simulink model "sampleModel1582_2"  (R2023a)
settings: Solver=VariableStepAuto  StartTime=0.0  StopTime=10.0  RelTol=1e-3
libraries: simulink x4, hdlsllib x1
settings Model: Creator=user1  LastModifiedBy=user1

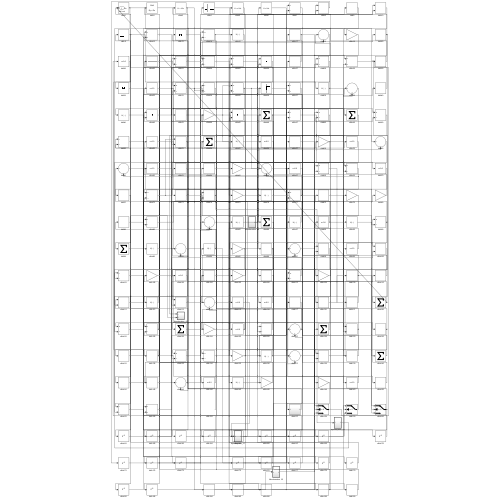
[thumbnail: Simulink's stored preview of the top-level diagram]
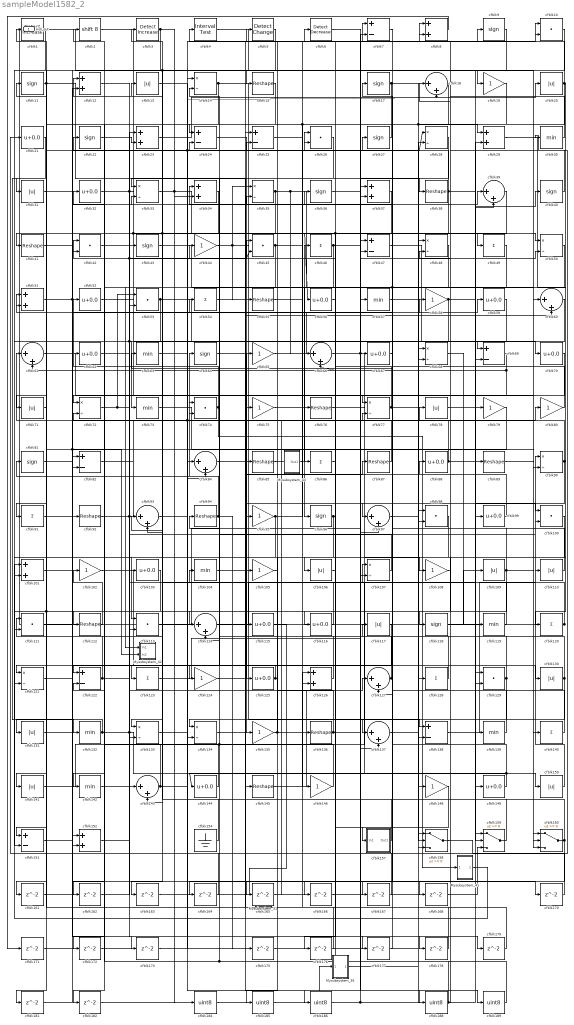
== system sampleModel1582_2 ==
  Mysubsystem_31 : Subsystem  TreatAsAtomicUnit=on  RTWFcnName=Mysubsystem_31
      settings: RTWFcnNameOpts=User specified  RTWFileNameOpts=Use function name
  Mysubsystem_35 : Subsystem  TreatAsAtomicUnit=on  RTWFcnName=Mysubsystem_35
      settings: RTWFcnNameOpts=User specified  RTWFileNameOpts=Use function name
  Mysubsystem_41 : Subsystem  TreatAsAtomicUnit=on  RTWFcnName=Mysubsystem_41
      settings: RTWFcnNameOpts=User specified  RTWFileNameOpts=Use function name
  Mysubsystem_42 : Subsystem  TreatAsAtomicUnit=on  RTWFcnName=Mysubsystem_42
      settings: RTWFcnNameOpts=User specified  RTWFileNameOpts=Use function name
  Mysubsystem_44 : Subsystem  TreatAsAtomicUnit=on  RTWFcnName=Mysubsystem_44
      settings: RTWFcnNameOpts=User specified  RTWFileNameOpts=Use function name
  cfblk1 : simulink/Logic and Bit Operations/Detect Increase  vinit=0.0  OutDataTypeStr=uint8
      settings: LibrarySourceBlock=|
      | hdlsllib/Logic and Bit
      | Operations/Detect
      | Increase
  cfblk{10,26,42,45,53,74,98,100,111,113,129} (11 alike) : DotProduct  OutDataTypeStr=uint8
  cfblk{8,12,23,29,34,37,51,101,126,152} (10 alike) : Sum  OutDataTypeStr=uint8
  cfblk{19,44,58,65,75,79..80,95,102,105,108,124,135,146,148} (15 alike) : Gain  OutDataTypeStr=uint8
  cfblk{21,32,52,56,59,62,67,70,88,99,103,115..116,125,144,149} (16 alike) : Bias  Bias=0.0  SaturateOnIntegerOverflow=off
  cfblk{30,57,63,73,104,119,132,139,142} (9 alike) : MinMax  OutDataTypeStr=uint8
  cfblk{13,20,31,71,78,106,109..110,117,130..131,141,150} (13 alike) : Abs  OutDataTypeStr=uint8  SaturateOnIntegerOverflow=off
  cfblk{14,28,33,35,48,50,68,72,77,90,107,121,133..134} (14 alike) : Product  Inputs=*/  OutDataTypeStr=uint8  RndMeth=Zero  SaturateOnIntegerOverflow=on
  cfblk{9,11,17,22,27,36,40,43,64,81,96,118} (12 alike) : Signum
  cfblk{15,38,41,55,76,85,87,89,92,94,112,136,145} (13 alike) : Reshape
  cfblk{18,39,60..61,66,84,93,97,114,127,137,143} (12 alike) : Sum  Inputs=|++  OutDataTypeStr=uint8
  cfblk{46,49,54,86,91,120,123,128,140} (9 alike) : Sum  Inputs=+  OutDataTypeStr=uint8
  cfblk{7,24..25,47,69,82,122,138,151} (9 alike) : Sum  Inputs=+-  OutDataTypeStr=uint8
  cfblk154 : Ground
  cfblk157 : Subsystem
      settings: LibrarySourceBlock=|
      | hdlsllib/Ports &
      | Subsystems/Subsystem
  cfblk158 : Switch  OutDataTypeStr=uint8  SaturateOnIntegerOverflow=off  InputSameDT=off
  cfblk159 : Switch  OutDataTypeStr=uint8  SaturateOnIntegerOverflow=off  InputSameDT=off
  cfblk160 : Switch  OutDataTypeStr=uint8  SaturateOnIntegerOverflow=off  InputSameDT=off
  cfblk{161..168,170..173,175..179,181..182} (19 alike) : Delay  SampleTime=1
  cfblk{184..186,188..189} (5 alike) : DataTypeConversion  OutDataTypeStr=uint8  SaturateOnIntegerOverflow=off  RndMeth=Floor
  cfblk2 : ArithShift  BitShiftNumber=8
  cfblk3 : simulink/Logic and Bit Operations/Detect Increase  vinit=0.0  OutDataTypeStr=uint8
      settings: LibrarySourceBlock=|
      | hdlsllib/Logic and Bit
      | Operations/Detect
      | Increase
  cfblk4 : hdlsllib/Logic and Bit Operations/Interval Test  IntervalClosedRight=on  uplimit=0.5  IntervalClosedLeft=on  lowlimit=-0.5  OutDataTypeStr=uint8
  cfblk5 : simulink/Logic and Bit Operations/Detect Change  vinit=0  OutDataTypeStr=uint8
      settings: LibrarySourceBlock=|
      | hdlsllib/Logic and Bit
      | Operations/Detect
      | Change
  cfblk6 : simulink/Logic and Bit Operations/Detect Decrease  vinit=0.0  OutDataTypeStr=uint8
      settings: LibrarySourceBlock=|
      | hdlsllib/Logic and Bit
      | Operations/Detect
      | Decrease
  Hdl_out : Outport  OutDataTypeStr=uint8
  wires:
  cfblk66/1 -> cfblk150/1, cfblk90/2
  cfblk60/1 -> cfblk73/1
  cfblk126/1 -> cfblk81/1
  cfblk47/1 -> cfblk70/1
  cfblk96/1 -> cfblk134/1, cfblk121/2
  cfblk21/1 -> cfblk132/1
  cfblk76/1 -> cfblk108/1
  cfblk14/1 -> cfblk138/1, cfblk172/1
  cfblk72/1 -> cfblk77/1, cfblk53/1
  cfblk118/1 -> cfblk109/1
  cfblk94/1 -> cfblk64/1, cfblk175/1
  cfblk49/1 -> cfblk96/1
  cfblk77/1 -> cfblk42/1, cfblk129/2
  cfblk31/1 -> cfblk92/1
  cfblk129/1 -> cfblk26/2, cfblk165/1
  cfblk92/1 -> cfblk47/1, cfblk80/1
  cfblk2/1 -> cfblk69/1
  cfblk146/1 -> cfblk94/1, cfblk2/1
  cfblk117/1 -> cfblk123/1
  cfblk74/1 -> Mysubsystem_41/1(In1), cfblk52/1
  cfblk24/1 -> cfblk135/1
  cfblk140/1 -> cfblk77/2
  cfblk131/1 -> cfblk27/1
  cfblk154/1 -> cfblk111/1
  cfblk71/1 -> cfblk141/1
  cfblk51/1 -> cfblk33/2, cfblk173/1
  cfblk95/1 -> cfblk151/1, cfblk8/2
  cfblk112/1 -> cfblk102/1
  cfblk56/1 -> cfblk116/1
  cfblk148/1 -> cfblk21/1
  cfblk29/1 -> cfblk118/1
  cfblk38/1 -> cfblk100/1, cfblk11/1, cfblk161/1
  cfblk135/1 -> cfblk47/2, cfblk115/1
  cfblk63/1 -> cfblk28/1, cfblk18/2
  cfblk18/1 -> cfblk126/2, cfblk71/1
  cfblk159/1 -> cfblk93/1
  cfblk57/1 -> cfblk158/1
  cfblk68/1 -> cfblk89/1
  cfblk110/1 -> cfblk51/1
  cfblk132/1 -> cfblk159/2, cfblk100/2, cfblk131/1
  cfblk124/1 -> cfblk65/1
  cfblk30/1 -> cfblk15/1
  cfblk53/1 -> cfblk101/2, cfblk133/2, cfblk75/1
  cfblk90/1 -> cfblk3/1, cfblk95/1
  cfblk7/1 -> cfblk97/1
  cfblk103/1 -> cfblk151/2, cfblk181/1
  cfblk101/1 -> cfblk125/1
  cfblk113/1 -> cfblk10/1
  cfblk73/1 -> cfblk97/2
  cfblk138/1 -> cfblk90/1
  cfblk32/1 -> cfblk86/1, cfblk69/2, cfblk177/1
  cfblk137/1 -> cfblk128/1
  cfblk37/1 -> cfblk72/1, cfblk103/1
  cfblk120/1 -> cfblk107/1, Hdl_out/1
  cfblk149/1 -> cfblk144/1, cfblk34/1
  cfblk1/1 -> cfblk111/2, cfblk39/2
  cfblk93/1 -> cfblk84/2
  cfblk15/1 -> cfblk112/1
  cfblk39/1 -> cfblk56/1, cfblk66/2
  cfblk3/1 -> cfblk41/1, cfblk184/1
  cfblk28/1 -> cfblk143/2
  cfblk25/1 -> cfblk76/1
  cfblk116/1 -> cfblk54/1
  cfblk43/1 -> cfblk149/1
  cfblk157/1(Out1) -> cfblk12/1
  cfblk150/1 -> cfblk110/1
  cfblk158/1 -> cfblk30/1
  cfblk23/1 -> cfblk20/1
  cfblk102/1 -> cfblk148/1
  cfblk45/1 -> Mysubsystem_42/1(In1), cfblk68/2
  cfblk80/1 -> cfblk17/1
  cfblk26/1 -> cfblk114/1
  cfblk141/1 -> cfblk79/1
  cfblk17/1 -> cfblk42/2, cfblk29/1
  cfblk67/1 -> cfblk137/1
  cfblk145/1 -> cfblk67/1
  cfblk35/1 -> cfblk160/1, cfblk66/1, cfblk113/2
  cfblk78/1 -> cfblk129/1
  cfblk59/1 -> cfblk152/2
  cfblk122/1 -> cfblk105/1, cfblk51/2
  cfblk98/1 -> cfblk185/1
  cfblk36/1 -> cfblk38/1
  cfblk86/1 -> cfblk106/1
  cfblk128/1 -> cfblk117/1
  cfblk22/1 -> cfblk23/2
  cfblk107/1 -> cfblk44/1
  cfblk6/1 -> cfblk188/1
  cfblk142/1 -> cfblk26/1, cfblk45/2
  cfblk139/1 -> cfblk63/1
  cfblk62/1 -> cfblk39/1
  cfblk87/1 -> cfblk74/1
  cfblk89/1 -> cfblk160/2
  cfblk65/1 -> cfblk58/1
  cfblk40/1 -> cfblk8/1
  cfblk12/1 -> cfblk43/1
  cfblk61/1 -> cfblk140/1
  cfblk11/1 -> cfblk145/1, cfblk31/1
  cfblk34/1 -> cfblk133/1
  cfblk64/1 -> cfblk7/1
  cfblk143/1 -> cfblk36/1, cfblk122/2
  cfblk4/1 -> cfblk60/1
  cfblk33/1 -> cfblk50/1, cfblk34/2
  cfblk27/1 -> cfblk24/1
  cfblk144/1 -> cfblk22/1
  cfblk127/1 -> cfblk157/1(In1), cfblk104/1
  cfblk9/1 -> cfblk33/1
  cfblk97/1 -> cfblk68/1
  cfblk50/1 -> cfblk166/1, cfblk167/1
  cfblk152/1 -> cfblk127/1
  cfblk119/1 -> cfblk13/1
  cfblk88/1 -> cfblk61/1, cfblk119/1
  cfblk5/1 -> cfblk82/2, cfblk163/1
  cfblk81/1 -> Mysubsystem_42/2(In2), cfblk62/1
  cfblk109/1 -> cfblk160/3, cfblk35/2, cfblk182/1
  cfblk160/1 -> cfblk78/1, cfblk164/1
  cfblk133/1 -> cfblk10/2
  cfblk55/1 -> cfblk130/1
  cfblk123/1 -> cfblk57/1
  cfblk111/1 -> cfblk59/1
  cfblk46/1 -> cfblk49/1, cfblk124/1
  cfblk44/1 -> cfblk139/1, cfblk35/1, cfblk55/1
  cfblk10/1 -> cfblk19/1
  cfblk75/1 -> cfblk146/1
  cfblk105/1 -> cfblk5/1
  cfblk79/1 -> cfblk91/1
  cfblk130/1 -> cfblk138/2, cfblk48/2
  cfblk52/1 -> cfblk136/1
  cfblk114/1 -> cfblk99/1
  cfblk100/1 -> cfblk113/1
  cfblk99/1 -> cfblk85/1
  cfblk48/1 -> cfblk142/1
  cfblk58/1 -> cfblk40/1, cfblk93/2
  cfblk85/1 -> cfblk9/1
  cfblk136/1 -> cfblk50/2, cfblk25/2
  cfblk20/1 -> cfblk158/2, cfblk53/2, cfblk120/1, cfblk4/1
  cfblk70/1 -> cfblk122/1
  cfblk121/1 -> cfblk74/2
  cfblk134/1 -> cfblk60/2
  cfblk42/1 -> cfblk24/2
  cfblk108/1 -> cfblk88/1
  cfblk125/1 -> cfblk45/1, cfblk121/1
  cfblk69/1 -> cfblk134/2, cfblk61/2
  cfblk82/1 -> cfblk7/2, cfblk14/1
  cfblk104/1 -> cfblk87/1
  cfblk161/1 -> cfblk143/1
  cfblk19/1 -> cfblk162/1
  cfblk162/1 -> cfblk23/1
  cfblk163/1 -> cfblk107/2
  cfblk164/1 -> cfblk82/1
  cfblk165/1 -> cfblk159/1
  cfblk166/1 -> cfblk28/2
  cfblk167/1 -> cfblk114/2
  cfblk41/1 -> cfblk168/1
  cfblk168/1 -> cfblk159/3
  cfblk151/1 -> cfblk170/1
  cfblk170/1 -> cfblk152/1
  cfblk8/1 -> cfblk171/1
  cfblk171/1 -> cfblk37/1
  cfblk172/1 -> cfblk158/3
  cfblk173/1 -> cfblk84/1
  cfblk175/1 -> cfblk137/2
  cfblk106/1 -> cfblk176/1
  cfblk176/1 -> cfblk25/1
  cfblk177/1 -> cfblk127/2
  cfblk54/1 -> cfblk178/1
  cfblk178/1 -> cfblk126/1
  cfblk91/1 -> cfblk179/1
  cfblk179/1 -> cfblk1/1
  cfblk181/1 -> cfblk12/2
  cfblk182/1 -> cfblk29/2
  cfblk185/1 -> cfblk48/1, cfblk37/2
  cfblk84/1 -> cfblk186/1
  cfblk186/1 -> cfblk98/1
  cfblk188/1 -> cfblk14/2, cfblk32/1, cfblk18/1
  cfblk13/1 -> cfblk189/1
  cfblk189/1 -> cfblk6/1
  cfblk115/1 -> Mysubsystem_31/1(In1)
  Mysubsystem_31/1(Out1) -> cfblk72/2
  cfblk184/1 -> Mysubsystem_35/1(In1)
  Mysubsystem_35/1(Out1) -> cfblk98/2
  Mysubsystem_41/1(Out1) -> cfblk101/1
  Mysubsystem_44/1(Out1) -> cfblk46/1

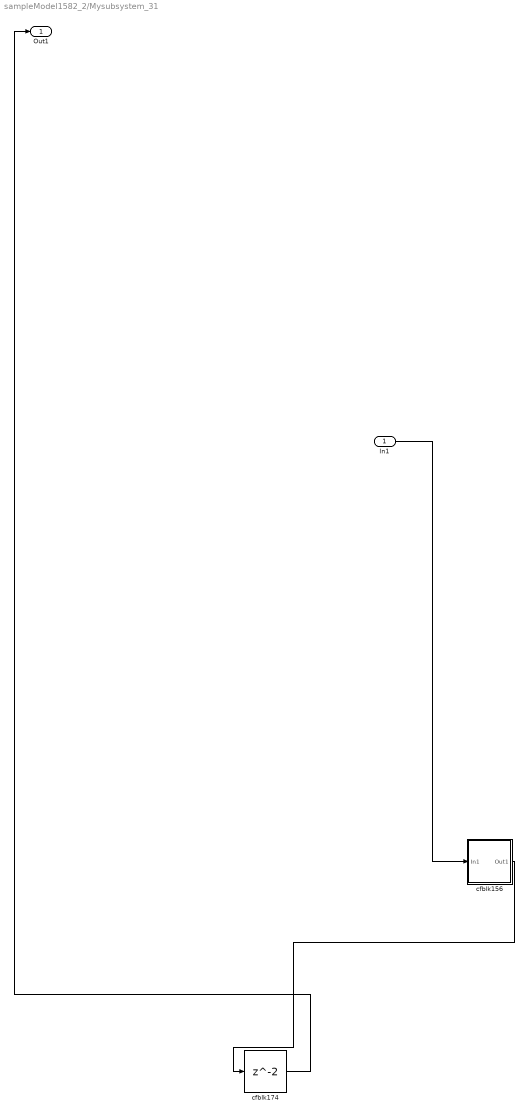
== system sampleModel1582_2/Mysubsystem_31 ==
  In1 : Inport
  cfblk156 : Subsystem
      settings: LibrarySourceBlock=|
      | hdlsllib/Ports &
      | Subsystems/Subsystem
  cfblk174 : Delay  SampleTime=1
  Out1 : Outport
  wires:
  cfblk156/1(Out1) -> cfblk174/1
  cfblk174/1 -> Out1/1
  In1/1 -> cfblk156/1(In1)

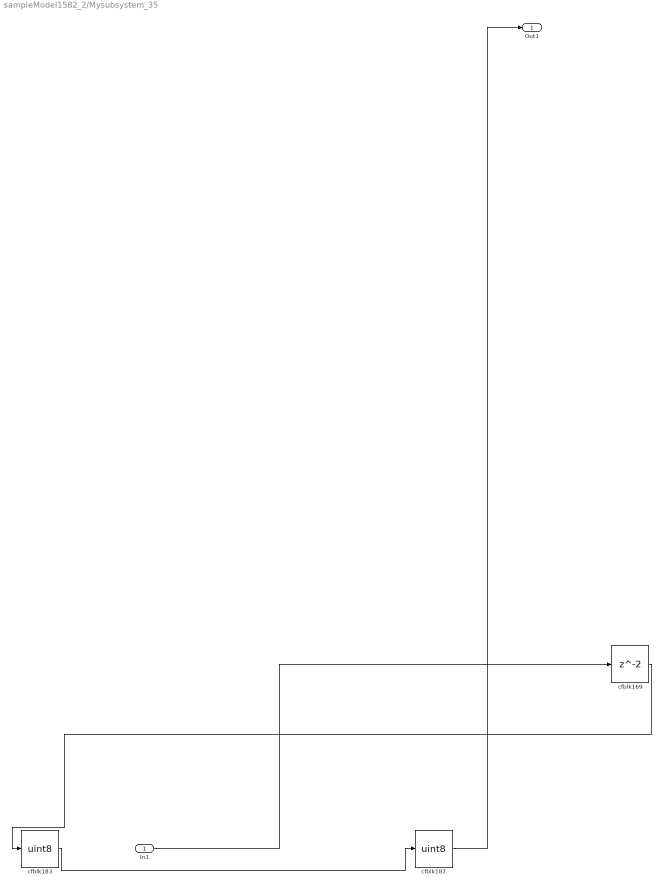
== system sampleModel1582_2/Mysubsystem_35 ==
  In1 : Inport
  cfblk169 : Delay  SampleTime=1
  cfblk183 : DataTypeConversion  OutDataTypeStr=uint8  SaturateOnIntegerOverflow=off  RndMeth=Floor
  cfblk187 : DataTypeConversion  OutDataTypeStr=uint8  SaturateOnIntegerOverflow=off  RndMeth=Floor
  Out1 : Outport
  wires:
  cfblk183/1 -> cfblk187/1
  In1/1 -> cfblk169/1
  cfblk169/1 -> cfblk183/1
  cfblk187/1 -> Out1/1

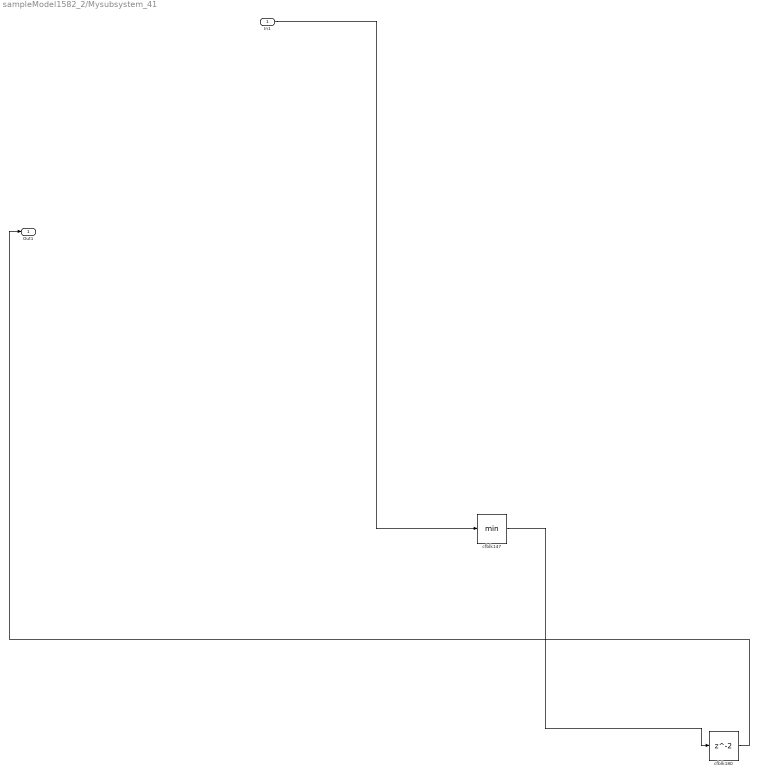
== system sampleModel1582_2/Mysubsystem_41 ==
  In1 : Inport
  cfblk147 : MinMax
  cfblk180 : Delay  SampleTime=1
  Out1 : Outport
  wires:
  cfblk147/1 -> cfblk180/1
  cfblk180/1 -> Out1/1
  In1/1 -> cfblk147/1

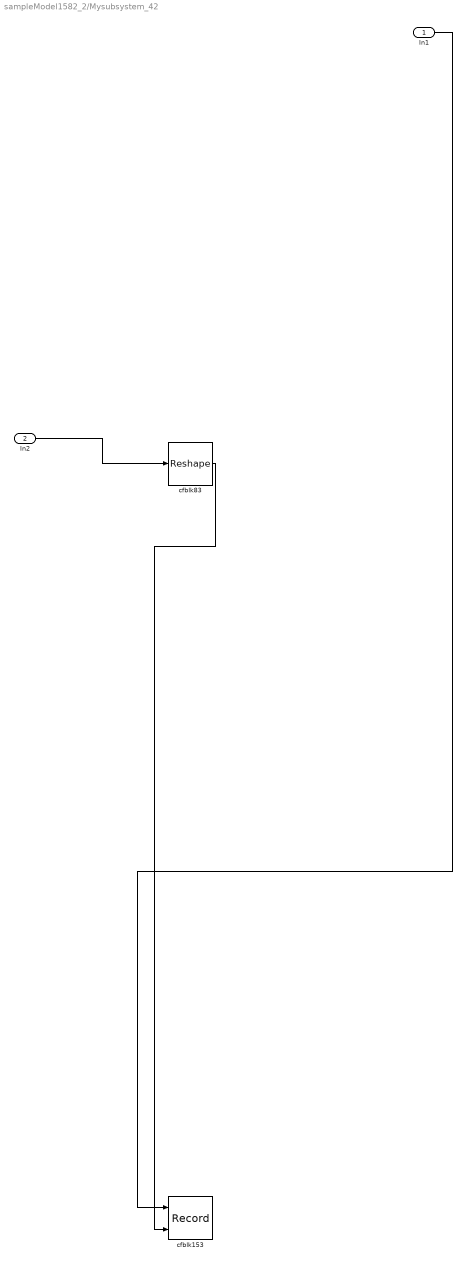
== system sampleModel1582_2/Mysubsystem_42 ==
  In1 : Inport
  In2 : Inport  Port=2
  cfblk153 : Record  FileSettingsInternal="{\"entries\":[{\"content\":{\"excelSettings\":{\"content\":{},\"type\":\"Streamout.ExcelSettings\"}},\"type\":\"Streamout.FileSettingStorage\",\"uuid\":\"\"}],\"packageUris\":[\"http:\\/\\/schema.mathworks.com\\/mf0\\/streamout_blocks\\/R2020a\"],\"version\":\"1.0\"}"  Layout=[1 1]  SignalsInternal="{\"entries\":[{\"content\":{},\"type\":\"RecordBlkView.InputSignals\",\"uuid\":\"\"}],\"packageUris\":[\"http:\\/\\/schema.mathworks.com\\/mf0\\/streamout_blocks\\/R2020a\"],\"version\":\"1.0\"}"  VisualizationBindings="{\"xyplotplugin\":{\"info\":[{\"series\":[],\"subplotID\":1}]}}"  CompatibilityTag=XY  st=-1
  cfblk83 : Reshape
  wires:
  cfblk83/1 -> cfblk153/2
  In2/1 -> cfblk83/1
  In1/1 -> cfblk153/1

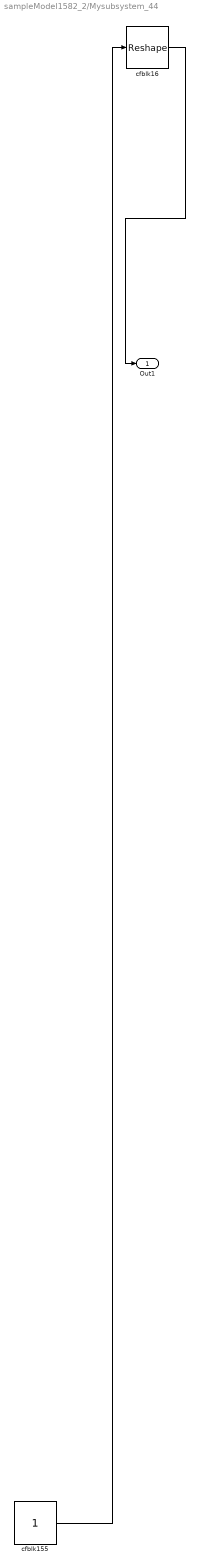
== system sampleModel1582_2/Mysubsystem_44 ==
  cfblk155 : Constant  SampleTime=-1
  cfblk16 : Reshape
  Out1 : Outport
  wires:
  cfblk16/1 -> Out1/1
  cfblk155/1 -> cfblk16/1

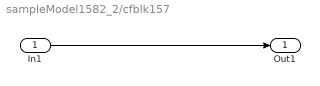
== system sampleModel1582_2/cfblk157 ==
  In1 : Inport
  Out1 : Outport
  wires:
  In1/1 -> Out1/1

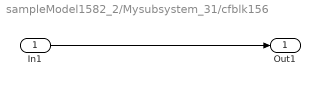
== system sampleModel1582_2/Mysubsystem_31/cfblk156 ==
  In1 : Inport
  Out1 : Outport
  wires:
  In1/1 -> Out1/1
